simulink model "sampleModel22"  (R2021b)
settings: Solver=VariableStepAuto  StartTime=0.0  StopTime=10.0  RelTol=1e-3
undefined symbols (not defined in the file or in its folder): Newton, Raphson
libraries: simulink x12, slpidlib x1
settings Model: Creator=user  LastModifiedBy=user

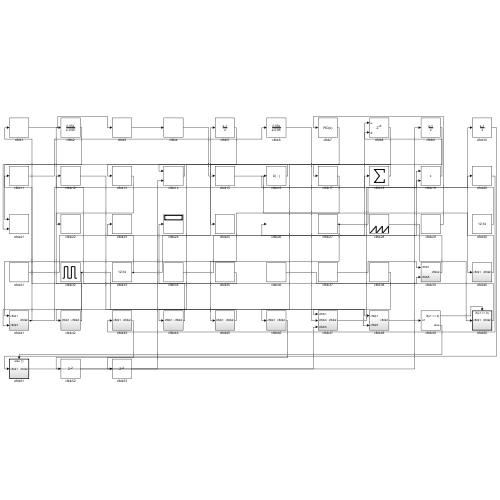
[thumbnail: Simulink's stored preview of the top-level diagram]
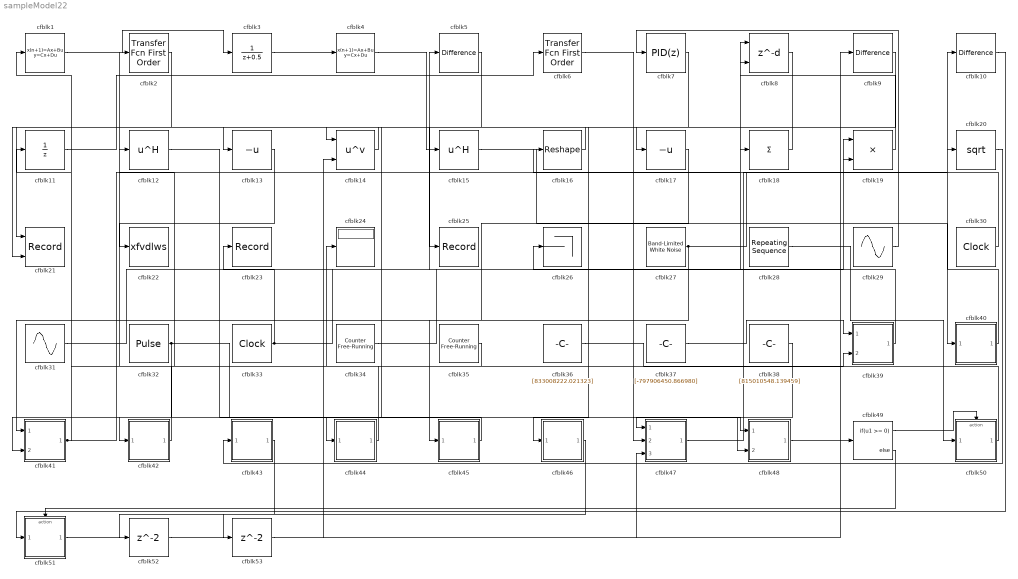
== system sampleModel22 ==
  cfblk1 : DiscreteStateSpace
  cfblk10 : simulink/Discrete/Difference  ICPrevInput=0.0  OutMin=[]  OutMax=[]  OutDataTypeStr=Inherit: Inherit via back propagation  OutDataType=fixdt(1, 16)  OutScaling=2^-10  DoSatur=off
  cfblk11 : UnitDelay  HasFrameUpgradeWarning=on
  cfblk12 : Math  Operator=hermitian  SaturateOnIntegerOverflow=on
  cfblk13 : UnaryMinus
  cfblk14 : Math  Operator=pow  SaturateOnIntegerOverflow=on
  cfblk15 : Math  Operator=hermitian  SaturateOnIntegerOverflow=on
  cfblk16 : Reshape
  cfblk17 : UnaryMinus
  cfblk18 : Sum  Inputs=+
  cfblk19 : Product  Inputs=**
  cfblk2 : simulink/Discrete/Transfer Fcn First Order  PoleZ=0.95  ICPrevOutput=0.0  DoSatur=off
  cfblk20 : Sqrt  SaturateOnIntegerOverflow=on
  cfblk21 : Record  FileSettingsInternal="{\"entries\":[{\"content\":{\"excelSettings\":{\"content\":{},\"type\":\"Streamout.ExcelSettings\"}},\"type\":\"Streamout.FileSettingStorage\",\"uuid\":\"d347088c-f2a3-4774-acaa-905cd5588dd1\"}],\"packageUris\":[\"http://schema.mathworks.com/mf0/streamout_blocks/R2020a\"],\"version\":\"1.0\"}"  Layout=[1 1]  SignalsInternal="{\"entries\":[{\"content\":{\"signals\":[{\"content\":{\"blockPath\":[\"sampleModel22/cfblk21\"],\"channel\":[],\"dimensions\":[1],\"domain\":\"sampleModel22/cfblk21\",\"lineColor\":\"#a2142f\",\"plots\":[1],\"port\":1,\"sid\":[\"\"],\"signalID\":900,\"signalName\":\"cfblk2\"},\"type\":\"RecordBlkView.Signal\",\"uuid\":\"72cce9bf-5026-4949-b22a-9a70ffc16a04\"},{\"content\":{\"blockPath\":[\"sampleModel22/cfblk21\"],\"channel\":[],\"dimensions\":[1],\"domain\":\"sampleModel22/cfblk21\",\"lineColor\":\"#139fff\",\"plots\":[1],\"port\":2,\"sid\":[\"\"],\"signalID\":904,\"signalName\":\"cfblk7\"},\"type\":\"RecordBlkView.Signal\",\"uuid\":\"bea1f47c-6652-4983-8379-7ae93b6d0a7d\"}]},\"type\":\"RecordBlkView.InputSignals\",\"uuid\":\"a3b7c627-b13b-45f5-a77d-88219f6db1f3\"}],\"packageUris\":[\"http://schema.mathworks.com/mf0/streamout_blocks/R2020a\"],\"version\":\"1.0\"}"  VisualizationBindings="{\"xyplotplugin\":{\"info\":[{\"series\":[{\"bindingParametersList\":[{\"parameter\":\"X-Axis\",\"signalID\":900,\"signalName\":\"cfblk2\"},{\"parameter\":\"Y-Axis\",\"signalID\":904,\"signalName\":\"cfblk7\"}],\"seriesID\":42425}],\"subplotID\":1}]}}"  CompatibilityTag=XY
  cfblk22 : ToWorkspace  VariableName=xfvdlws  SaveFormat=Timeseries  SampleTime=-1
  cfblk23 : Record  FileSettingsInternal="{\"entries\":[{\"content\":{\"excelSettings\":{\"content\":{},\"type\":\"Streamout.ExcelSettings\"}},\"type\":\"Streamout.FileSettingStorage\",\"uuid\":\"aba5f315-0ffa-4260-b08e-6ada968d828a\"}],\"packageUris\":[\"http://schema.mathworks.com/mf0/streamout_blocks/R2020a\"],\"version\":\"1.0\"}"  SignalsInternal="{\"entries\":[{\"content\":{\"signals\":[{\"content\":{\"blockPath\":[\"sampleModel22/cfblk23\"],\"channel\":[],\"dimensions\":[1],\"domain\":\"sampleModel22/cfblk23\",\"lineColor\":\"#64d413\",\"plots\":[1],\"port\":1,\"sid\":[\"\"],\"signalID\":908,\"signalName\":\"cfblk33\"},\"type\":\"RecordBlkView.Signal\",\"uuid\":\"00477b48-f975-47f7-aa1d-9a892664fb2a\"}]},\"type\":\"RecordBlkView.InputSignals\",\"uuid\":\"32843abc-300b-4a92-8da5-51a580ef2afe\"}],\"packageUris\":[\"http://schema.mathworks.com/mf0/streamout_blocks/R2020a\"],\"version\":\"1.0\"}"  VisualizationBindings="{\"sparklinesplugin\":{\"info\":[{\"bindingParametersList\":[],\"subplotID\":1}]}}"
  cfblk24 : Display
  cfblk25 : Record  FileSettingsInternal="{\"entries\":[{\"content\":{\"excelSettings\":{\"content\":{},\"type\":\"Streamout.ExcelSettings\"}},\"type\":\"Streamout.FileSettingStorage\",\"uuid\":\"a09df4a2-82cf-4162-b1e9-cd908c00b4bb\"}],\"packageUris\":[\"http://schema.mathworks.com/mf0/streamout_blocks/R2020a\"],\"version\":\"1.0\"}"  SignalsInternal="{\"entries\":[{\"content\":{\"signals\":[{\"content\":{\"blockPath\":[\"sampleModel22/cfblk25\"],\"channel\":[],\"dimensions\":[1],\"domain\":\"sampleModel22/cfblk25\",\"lineColor\":\"#ff13a6\",\"plots\":[1],\"port\":1,\"sid\":[\"\"],\"signalID\":912,\"signalName\":\"cfblk5\"},\"type\":\"RecordBlkView.Signal\",\"uuid\":\"83a76baf-6ea0-4cc0-9cd0-b4f16879e093\"}]},\"type\":\"RecordBlkView.InputSignals\",\"uuid\":\"d9d92264-43dd-4799-a9ea-abcf50968a61\"}],\"packageUris\":[\"http://schema.mathworks.com/mf0/streamout_blocks/R2020a\"],\"version\":\"1.0\"}"  VisualizationBindings="{\"sparklinesplugin\":{\"info\":[{\"bindingParametersList\":[],\"subplotID\":1}]}}"
  cfblk26 : Terminator
  cfblk27 : simulink/Sources/Band-Limited White Noise  Cov=[4970221828.637503]  Ts=0.1  seed=[6095968655.000000]
  cfblk28 : simulink/Sources/Repeating Sequence  rep_seq_t=[0 2]  rep_seq_y=[-844343196.822376, -517134607.441351]
  cfblk29 : Sin  Amplitude=[-948431688.326203]  Bias=[692953871.845322]  SampleTime=0
  cfblk3 : DiscreteTransferFcn  SampleTime=1
  cfblk30 : DigitalClock
  cfblk31 : Sin  Amplitude=[-970274407.735577]  Bias=[100831776.825705]  SampleTime=0
  cfblk32 : DiscretePulseGenerator  PulseType=Time based  Amplitude=[-760657684.991832]  Period=[58794913.073271]  PulseWidth=5  PhaseDelay=[6.000000]
  cfblk33 : DigitalClock
  cfblk34 : simulink/Sources/Counter Free-Running  NumBits=[45.000000]  tsamp=-1
  cfblk35 : simulink/Sources/Counter Free-Running  NumBits=[19.000000]  tsamp=-1
  cfblk36 : Constant  Value=[833008222.021323]  SampleTime=1
  cfblk37 : Constant  Value=[-797906450.866980]  SampleTime=1
  cfblk38 : Constant  Value=[815010548.139459]  SampleTime=1
  cfblk39 : Subsystem
  cfblk4 : DiscreteStateSpace
  cfblk40 : Subsystem
  cfblk41 : Subsystem
  cfblk42 : Subsystem
  cfblk43 : Subsystem
  cfblk44 : Subsystem
  cfblk45 : Subsystem
  cfblk46 : Subsystem
  cfblk47 : Subsystem
  cfblk48 : Subsystem
  cfblk49 : If  IfExpression=u1 >= 0  SampleTime=1
  cfblk5 : simulink/Discrete/Difference  ICPrevInput=0.0  OutMin=[]  OutMax=[]  OutDataTypeStr=Inherit: Inherit via back propagation  OutDataType=fixdt(1, 16)  OutScaling=2^-10  DoSatur=off
  cfblk50 : Subsystem  TreatAsAtomicUnit=on
  cfblk51 : Subsystem  TreatAsAtomicUnit=on
  cfblk52 : Delay  SampleTime=1
  cfblk53 : Delay  SampleTime=1
  cfblk6 : simulink/Discrete/Transfer Fcn First Order  PoleZ=0.95  ICPrevOutput=0.0  DoSatur=off
  cfblk7 : slpidlib/PID Controller  Controller=PID  Form=Parallel  TimeDomain=Discrete-time  UseExternalTs=off  SampleTime=1  IntegratorMethod=Forward Euler  FilterMethod=Forward Euler  ControllerParametersSource=internal  P=1  I=1  D=0  UseFilter=on  N=100  TunerSelectOption=Transfer Function Based (PID Tuner App)  InitialConditionSource=internal  InitialConditionForIntegrator=0  InitialConditionForFilter=0  DifferentiatorICPrevScaledInput=0  ExternalReset=none  TrackingMode=off  Kt=1  LimitOutput=off  SatLimitsSource=internal  UpperSaturationLimit=inf  LowerSaturationLimit=-inf  LinearizeAsGain=off  AntiWindupMode=none  Kb=1  POutMin=[]  POutMax=[]  IOutMin=[]  IOutMax=[]  DOutMin=[]  DOutMax=[]  NOutMin=[]  NOutMax=[]  SumOutMin=[]  SumOutMax=[]  SaturationOutMin=[]  SaturationOutMax=[]  PParamMin=[]  PParamMax=[]  IParamMin=[]  IParamMax=[]  DParamMin=[]  DParamMax=[]  NParamMin=[]  NParamMax=[]  KbParamMin=[]  KbParamMax=[]  KtParamMin=[]  KtParamMax=[]  KbOutMin=[]  KbOutMax=[]  KtOutMin=[]  KtOutMax=[]  IntegratorOutMin=[]  IntegratorOutMax=[]  FilterOutMin=[]  FilterOutMax=[]  SumI1OutMin=[]  SumI1OutMax=[]  SumI2OutMin=[]  SumI2OutMax=[]  SumI3OutMin=[]  SumI3OutMax=[]  SumI4OutMin=[]  SumI4OutMax=[]  SumDOutMin=[]  SumDOutMax=[]  DifferentiatorOutMin=[]  DifferentiatorOutMax=[]  FilterDiffOutCoefMin=[]  FilterDiffOutCoefMax=[]  ReciprocalOutMin=[]  ReciprocalOutMax=[]  SumDenOutMin=[]  SumDenOutMax=[]  SumNumOutMin=[]  SumNumOutMax=[]  DivideOutMin=[]  DivideOutMax=[]  UdiffTsProdOutMin=[]  UdiffTsProdOutMax=[]  NTsProdOutMin=[]  NTsProdOutMax=[]  UintegralTsProdOutMin=[]  UintegralTsProdOutMax=[]  UngainTsProdOutMin=[]  UngainTsProdOutMax=[]  IntegratorContinuousStateAttributes=''  IntegratorStateMustResolveToSignalObject=off  IntegratorRTWStateStorageClass=Auto  FilterContinuousStateAttributes=''  FilterStateMustResolveToSignalObject=off  FilterRTWStateStorageClass=Auto  ParallelPVariant=InternalParameters  IdealPVariant=Disabled  IVariant=InternalParameters  DVariant=InternalParameters  IntegratorVariant=Discrete  SatVariant=Disabled  AWVariant=Passthrough  PCopyVariant=Disabled  TRVariant=Disabled  FdbkBlocksVariant=Forward  IdealPFdbkVariant=Disabled  SatFdbkVariant=Disabled  DerivativeFilterVariant=ForwardEulerFilter  NVariant=InternalParameters  NCopyVariant=Disabled  FilterICVariant=InternalICsFilter  IntegratorICVariant=InternalICs  ExternalResetVariant=Disabled  TRSumVariant=Passthrough  SumFdbkVariant=Disabled  SumVariant=Sum_PID  TsampFilterVariant=InternalTs  TsampNgainVariant=Passthrough  TsampIntegralVariant=Passthrough  ExternalSaturationOutDataTypeStr=Inherit: Same as second input
  cfblk8 : Delay  DelayLengthSource=Input port  SampleTime=1
      settings: InputPortMap=u0,p1
  cfblk9 : simulink/Discrete/Difference  ICPrevInput=0.0  OutMin=[]  OutMax=[]  OutDataTypeStr=Inherit: Inherit via back propagation  OutDataType=fixdt(1, 16)  OutScaling=2^-10  DoSatur=off
  wires:
  cfblk38/1 -> cfblk47/1(cfblk1)
  cfblk39/1(cfblk2) -> cfblk26/1
  cfblk18/1 -> cfblk17/1
  cfblk48/1(cfblk2) -> cfblk49/1
  cfblk3/1 -> cfblk4/1
  cfblk29/1 -> cfblk7/1
  cfblk1/1 -> cfblk3/1
  cfblk33/1 -> cfblk5/1, cfblk23/1
  cfblk35/1 -> cfblk2/1
  cfblk5/1 -> cfblk25/1
  cfblk16/1 -> cfblk14/1
  cfblk40/1(cfblk2) -> cfblk10/1
  cfblk2/1 -> cfblk21/1
  cfblk45/1(cfblk2) -> cfblk42/1(cfblk1)
  cfblk42/1(cfblk2) -> cfblk11/1
  cfblk4/1 -> cfblk15/1
  cfblk50/1(cfblk2) -> cfblk24/1
  cfblk17/1 -> cfblk45/1(cfblk1)
  cfblk20/1 -> cfblk43/1(cfblk1)
  cfblk47/1(cfblk2) -> cfblk20/1
  cfblk37/1 -> cfblk39/1(cfblk1)
  cfblk8/1 -> cfblk44/1(cfblk1)
  cfblk15/1 -> cfblk40/1(cfblk1)
  cfblk31/1 -> cfblk8/1
  cfblk7/1 -> cfblk21/2
  cfblk13/1 -> cfblk22/1
  cfblk6/1 -> cfblk48/1(cfblk1)
  cfblk44/1(cfblk2) -> cfblk12/1
  cfblk14/1 -> cfblk13/1
  cfblk41/1(cfblk2) -> cfblk18/1, cfblk1/1
  cfblk36/1 -> cfblk39/2(cfblk5)
  cfblk11/1 -> cfblk6/1
  cfblk9/1 -> cfblk46/1(cfblk1)
  cfblk32/1 -> cfblk48/2(cfblk5), cfblk41/2(cfblk3)
  cfblk12/1 -> cfblk47/2(cfblk4)
  cfblk28/1 -> cfblk50/1(cfblk1)
  cfblk19/1 -> cfblk8/2
  cfblk30/1 -> cfblk16/1
  cfblk34/1 -> cfblk19/1
  cfblk10/1 -> cfblk51/1(cfblk1)
  cfblk51/1(cfblk2) -> cfblk14/2
  cfblk27/1 -> cfblk41/1(cfblk1), cfblk19/2
  cfblk49/1 -> cfblk50/Action
  cfblk49/2 -> cfblk51/Action
  cfblk43/1(cfblk2) -> cfblk52/1
  cfblk52/1 -> cfblk47/3(cfblk5)
  cfblk46/1(cfblk2) -> cfblk53/1
  cfblk53/1 -> cfblk9/1

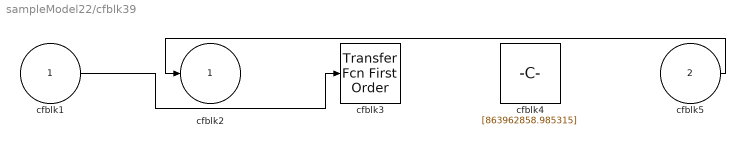
== system sampleModel22/cfblk39 ==
  cfblk1 : Inport
  cfblk5 : Inport  Port=2
  cfblk3 : simulink/Discrete/Transfer Fcn First Order  PoleZ=0.95  ICPrevOutput=0.0  DoSatur=off
  cfblk4 : Constant  Value=[863962858.985315]  SampleTime=1
  cfblk2 : Outport
  wires:
  cfblk5/1 -> cfblk2/1
  cfblk1/1 -> cfblk3/1

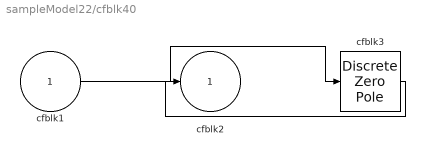
== system sampleModel22/cfblk40 ==
  cfblk1 : Inport
  cfblk3 : DiscreteZeroPole  Poles=[0 0.5]  Gain=1
  cfblk2 : Outport
  wires:
  cfblk1/1 -> cfblk3/1
  cfblk3/1 -> cfblk2/1

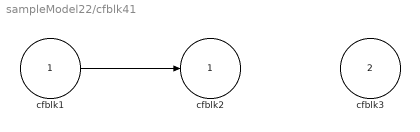
== system sampleModel22/cfblk41 ==
  cfblk1 : Inport
  cfblk3 : Inport  Port=2
  cfblk2 : Outport
  wires:
  cfblk1/1 -> cfblk2/1

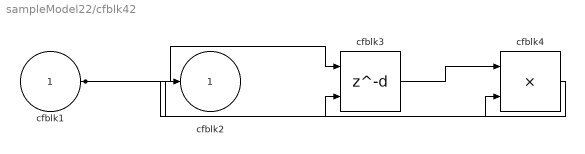
== system sampleModel22/cfblk42 ==
  cfblk1 : Inport
  cfblk3 : Delay  DelayLengthSource=Input port  SampleTime=1
      settings: InputPortMap=u0,p1
  cfblk4 : Product
  cfblk2 : Outport
  wires:
  cfblk1/1 -> cfblk3/1, cfblk4/2, cfblk3/2
  cfblk4/1 -> cfblk2/1
  cfblk3/1 -> cfblk4/1

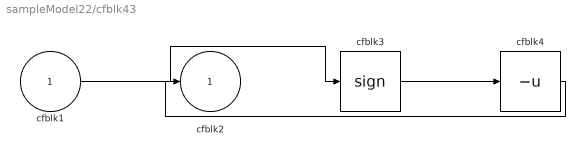
== system sampleModel22/cfblk43 ==
  cfblk1 : Inport
  cfblk3 : Signum
  cfblk4 : UnaryMinus
  cfblk2 : Outport
  wires:
  cfblk1/1 -> cfblk3/1
  cfblk3/1 -> cfblk4/1
  cfblk4/1 -> cfblk2/1

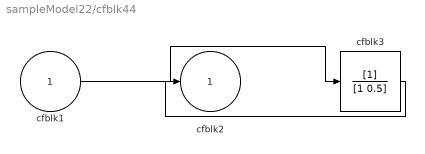
== system sampleModel22/cfblk44 ==
  cfblk1 : Inport
  cfblk3 : DiscreteFilter  SampleTime=1
  cfblk2 : Outport
  wires:
  cfblk1/1 -> cfblk3/1
  cfblk3/1 -> cfblk2/1

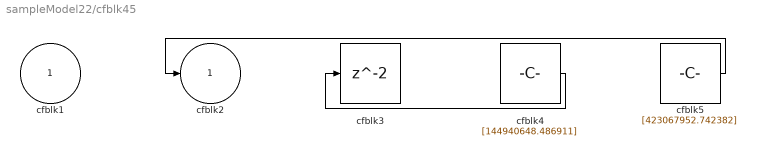
== system sampleModel22/cfblk45 ==
  cfblk1 : Inport
  cfblk3 : Delay  SampleTime=1
  cfblk4 : Constant  Value=[144940648.486911]  SampleTime=1
  cfblk5 : Constant  Value=[423067952.742382]  SampleTime=1
  cfblk2 : Outport
  wires:
  cfblk5/1 -> cfblk2/1
  cfblk4/1 -> cfblk3/1

== system sampleModel22/cfblk46 ==
  cfblk1 : Inport
  cfblk3 : UnaryMinus
  cfblk2 : Outport
  wires:
  cfblk1/1 -> cfblk2/1, cfblk3/1

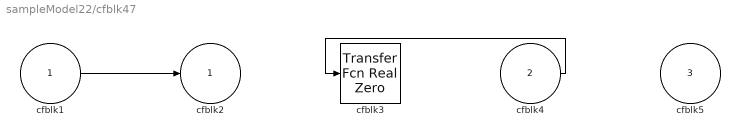
== system sampleModel22/cfblk47 ==
  cfblk1 : Inport
  cfblk4 : Inport  Port=2
  cfblk5 : Inport  Port=3
  cfblk3 : simulink/Discrete/Transfer Fcn Real Zero  ZeroZ=0.75  ICPrevInput=0.0  DoSatur=off
      settings: SourceProductBaseCode=SL
  cfblk2 : Outport
  wires:
  cfblk1/1 -> cfblk2/1
  cfblk4/1 -> cfblk3/1

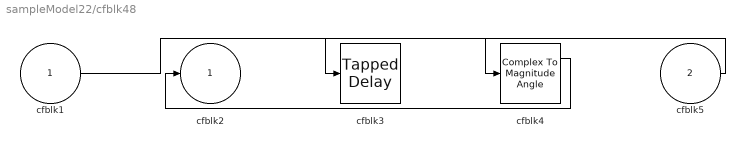
== system sampleModel22/cfblk48 ==
  cfblk1 : Inport
  cfblk5 : Inport  Port=2
  cfblk3 : simulink/Discrete/Tapped Delay  vinit=0.0  samptime=-1  NumDelays=1  DelayOrder=Oldest  includeCurrent=off
  cfblk4 : ComplexToMagnitudeAngle
  cfblk2 : Outport
  wires:
  cfblk5/1 -> cfblk3/1
  cfblk4/1 -> cfblk2/1
  cfblk1/1 -> cfblk4/1

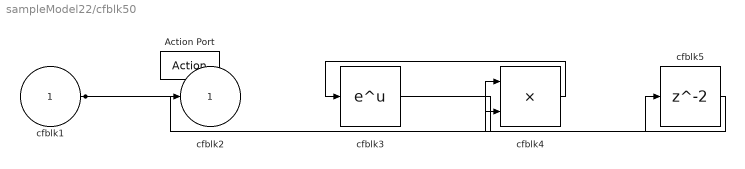
== system sampleModel22/cfblk50 ==
  cfblk1 : Inport
  Action Port : ActionPort  ActionPortLabel=if(u1 >= 0)
  cfblk3 : Math  SaturateOnIntegerOverflow=on
  cfblk4 : Product  Inputs=**
  cfblk5 : Delay
  cfblk2 : Outport
  wires:
  cfblk1/1 -> cfblk4/1, cfblk2/1
  cfblk4/1 -> cfblk3/1
  cfblk3/1 -> cfblk5/1
  cfblk5/1 -> cfblk4/2

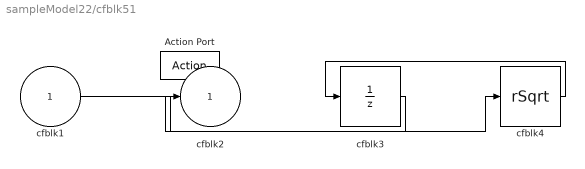
== system sampleModel22/cfblk51 ==
  cfblk1 : Inport
  Action Port : ActionPort  ActionPortLabel=else
  cfblk3 : UnitDelay  SampleTime=-1  HasFrameUpgradeWarning=on
  cfblk4 : Sqrt  Operator=rSqrt  AlgorithmType=Newton-Raphson  SaturateOnIntegerOverflow=on
  cfblk2 : Outport
  wires:
  cfblk4/1 -> cfblk3/1
  cfblk1/1 -> cfblk4/1
  cfblk3/1 -> cfblk2/1
